simulink model "SFC_graph"  (R2024b)
settings: Solver=VariableStepAuto  StartTime=0.0  StopTime=10.0  RelTol=1e-3
values from neighbouring files (symbols this model uses):
  K = PHT/(H_aux*PHT + diag(matR(ind_z)))    [EKF_IMU.m]    (also in EKF_NAV.m; EKF_WFL.m; PID_MV.m = PARAM.K; SFC.m = PARAM.K)
undefined symbols (not defined in the file or in its folder): u0, x0
libraries: simulink x1
settings Model: Creator=diego-ubuntu  LastModifiedBy=diego-ubuntu

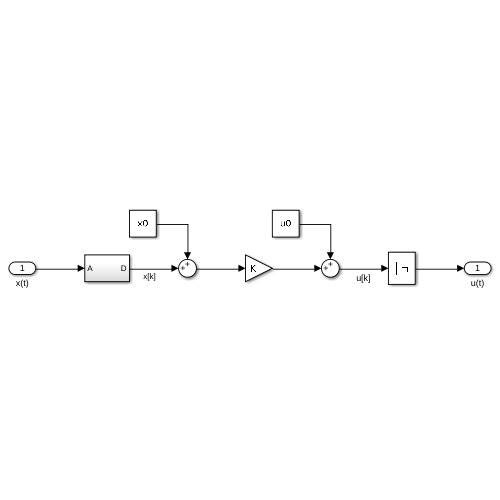
[thumbnail: Simulink's stored preview of the top-level diagram]
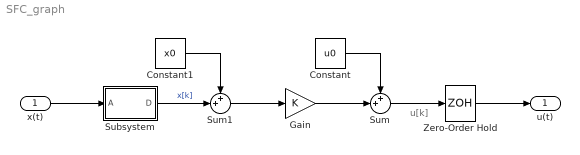
== system SFC_graph ==
  note: u[k]
  x(t) : Inport
  Constant : Constant  Value=u0
  Constant1 : Constant  Value=x0
  Gain : Gain  Gain=K
  Subsystem : Subsystem
  Sum : Sum  Inputs=++|
  Sum1 : Sum  Inputs=++|
  Zero-Order Hold : ZeroOrderHold  SampleTime=-1
  u(t) : Outport
  wires:
  Sum/1 -> Zero-Order Hold/1
  Gain/1 -> Sum/2
  Constant/1 -> Sum/1
  Constant1/1 -> Sum1/1
  Sum1/1 -> Gain/1
  Subsystem/1(D) -> Sum1/2  "x[k]"
  x(t)/1 -> Subsystem/1(A)
  Zero-Order Hold/1 -> u(t)/1

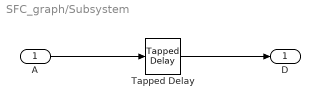
== system SFC_graph/Subsystem ==
  A : Inport
  Tapped Delay : simulink/Discrete/Tapped Delay  vinit=0.0  samptime=-1  NumDelays=4  DelayOrder=Oldest  includeCurrent=off
  D : Outport
  wires:
  A/1 -> Tapped Delay/1
  Tapped Delay/1 -> D/1
